simulink model "Model"  (R2023b)
settings: Solver=VariableStepAuto  StartTime=0.0  StopTime=10.0  RelTol=1e-3
libraries: simulink x1
settings Model: Creator=JesperBertelsen  LastModifiedBy=JesperBertelsen

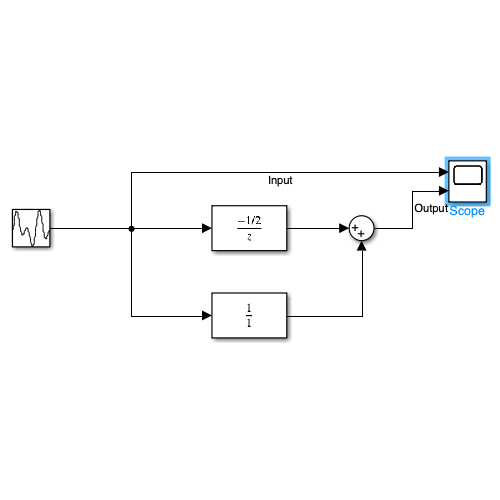
[thumbnail: Simulink's stored preview of the top-level diagram]
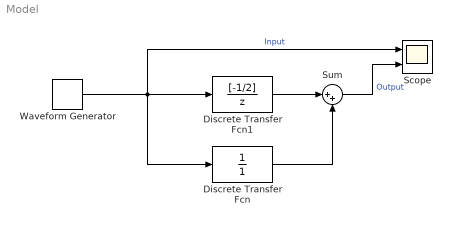
== system Model ==
  Discrete Transfer Fcn : DiscreteTransferFcn  Denominator=[1]
  Discrete Transfer Fcn1 : DiscreteTransferFcn  Numerator=[-1/2]  Denominator=[1 0]
  Scope : Scope  NumInputPorts=2
  Sum : Sum  Inputs=|++
  Waveform Generator : simulink/Sources/Waveform Generator  OutMin=[]  OutMax=[]  OutDataTypeStr=double  SelectedSignal=1  Signals=sin(1, pi/4, 90)  BlockNames=MultiportSwitch_9672a4fdef9a47c  SampleTime=0.1
  wires:
  Waveform Generator/1 -> Scope/1, Discrete Transfer Fcn1/1, Discrete Transfer Fcn/1  "Input"
  Discrete Transfer Fcn/1 -> Sum/2
  Discrete Transfer Fcn1/1 -> Sum/1
  Sum/1 -> Scope/2  "Output"
